simulink model "ep5_1"  (R2018a)
settings: Solver=VariableStepAuto  StartTime=0.0  StopTime=10.0  RelTol=1e-3
settings Model: Creator=zheny  LastModifiedBy=zheny

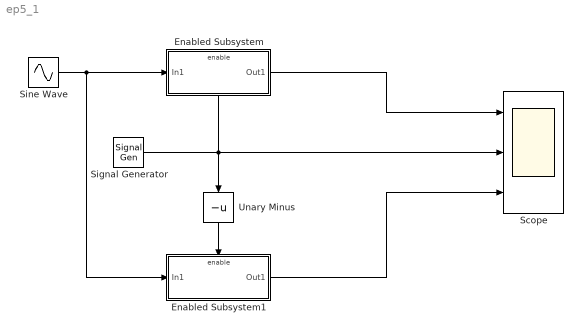
== system ep5_1 ==
  Enabled Subsystem : Subsystem  TreatAsAtomicUnit=on
  Enabled Subsystem1 : Subsystem  TreatAsAtomicUnit=on
  Scope : Scope  NumInputPorts=3
  Signal Generator : SignalGenerator  WaveForm=square
  Sine Wave : Sin  SampleTime=0
  Unary Minus : UnaryMinus
  wires:
  Sine Wave/1 -> Enabled Subsystem/1(In1), Enabled Subsystem1/1(In1)
  Enabled Subsystem/1(Out1) -> Scope/1
  Enabled Subsystem1/1(Out1) -> Scope/3
  Signal Generator/1 -> Unary Minus/1, Enabled Subsystem/Enable, Scope/2
  Unary Minus/1 -> Enabled Subsystem1/Enable

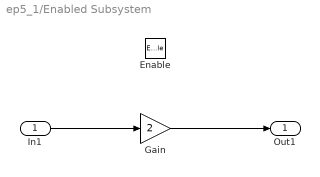
== system ep5_1/Enabled Subsystem ==
  In1 : Inport
  Enable : EnablePort  StatesWhenEnabling=reset
  Gain : Gain  Gain=2
  Out1 : Outport
  wires:
  In1/1 -> Gain/1
  Gain/1 -> Out1/1

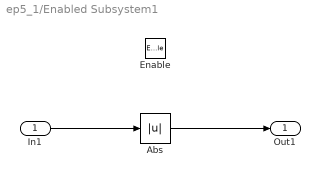
== system ep5_1/Enabled Subsystem1 ==
  In1 : Inport
  Enable : EnablePort
  Abs : Abs
  Out1 : Outport
  wires:
  In1/1 -> Abs/1
  Abs/1 -> Out1/1
